simulink model "tp_auto_model (1)"  (R2019a)
settings: Solver=FixedStepAuto  StartTime=0.0  StopTime=20  FixedStep=0.002  RelTol=1e-3  EnableMultiTasking=on
PostLoadFcn:
  | qc_set_target_type(getConfigSet(bdroot, 'QUARC Default Target Configuration'));
values from neighbouring files (symbols this model uses):
  A_c = Axo - L*C    [TP_AUTO_II.m]
  Axo = [ 0 0 1 0 ; 0 0 0 1 ; 0 149 -17 4.91 ; 0 -262 16.8 -8.61]    [TP_AUTO_II.m]
  B_c = [L  Bxo]    [TP_AUTO_II.m]
  Bxo = [0 ; 0 ; -49.7 ; 49.1]    [TP_AUTO_II.m]
  K1 = lqr(Axo , Bxo , Q1 , R)    [TP_AUTO_II.m]
undefined symbols (not defined in the file or in its folder): HIL
libraries: quarc_library x5, cstblocks x2, simulink x1
settings Model: ExtModeTrigDuration=10000  Creator=MLevis  LastModifiedBy=3700500
settings SolverCC: PositivePriorityOrder=on
settings DataIOCC: LimitDataPoints=on  SaveFormat=Array  SignalLoggingSaveFormat=ModelDataLogs  ReturnWorkspaceOutputs=off
settings OptimizationCC: ExpressionDepthLimit=2147483647  InitFltsAndDblsToZero=on  LifeSpan=inf
settings DebuggingCC: SaveWithParameterizedLinksMsg=none  UnderspecifiedInitializationDetection=Classic  MergeDetectMultiDrivingBlocksExec=none  SolverPrmCheckMsg=warning  MultiTaskDSMMsg=warning  MultiTaskCondExecSysMsg=none  FcnCallInpInsideContextMsg=warning  StateNameClashWarn=warning  SFUnexpectedBacktrackingDiag=warning  SFNoUnconditionalDefaultTransitionDiag=warning  SFExecutionAtInitializationDiag=none  ArithmeticOperatorsInVariantConditions=warning
settings HardwareCC: ProdBitPerPointer=32  ProdBitPerSizeT=32  ProdBitPerPtrDiffT=32  ProdLargestAtomicFloat=None  ProdIntDivRoundTo=Undefined  ProdEndianess=Unspecified  ProdWordSize=32  ProdHWDeviceType=32-bit Generic
settings ModelReferenceCC: PropagateSignalLabelsOutOfModel=off
settings SFSimCC: SimUseLocalCustomCode=off
settings RTWCC: SystemTargetFile=quarc_win64.tlc  TemplateMakefile=quarc_default_tmf  Description=QUARC Win64 Target  RTWUseLocalCustomCode=off
settings CodeAppCC: StateflowObjectComments=on
settings STFCustomTargetCC: TargetPreCompLibLocation=C:\PROGRA~3\QUARC\lib\2019a\win64\release  ConcurrentExecutionCompliant=on  GeneratePreprocessorConditionals=Disable all  CPPClassGenCompliant=on  SystemTargetFile=quarc_win64.tlc
settings GRTTargetCC: TargetPreCompLibLocation=C:\PROGRA~3\QUARC\lib\2019a\win64\release  TargetLangStandard=C89/C90 (ANSI)  ParMdlRefBuildCompliant=off  CompOptLevelCompliant=off  GeneratePreprocessorConditionals=Disable all  CombineOutputUpdateFcns=off  MatFileLogging=off  GRTInterface=on  UseToolchainInfoCompliant=off  ExtMode=on  ExtModeMexFile=quarc_comm
settings ConfigComp: CovMetricSettings=dw  CovHtmlReporting=on  CovSaveCumulativeToWorkspaceVar=on  CovSaveSingleToWorkspaceVar=on  CovExternalEMLEnable=off

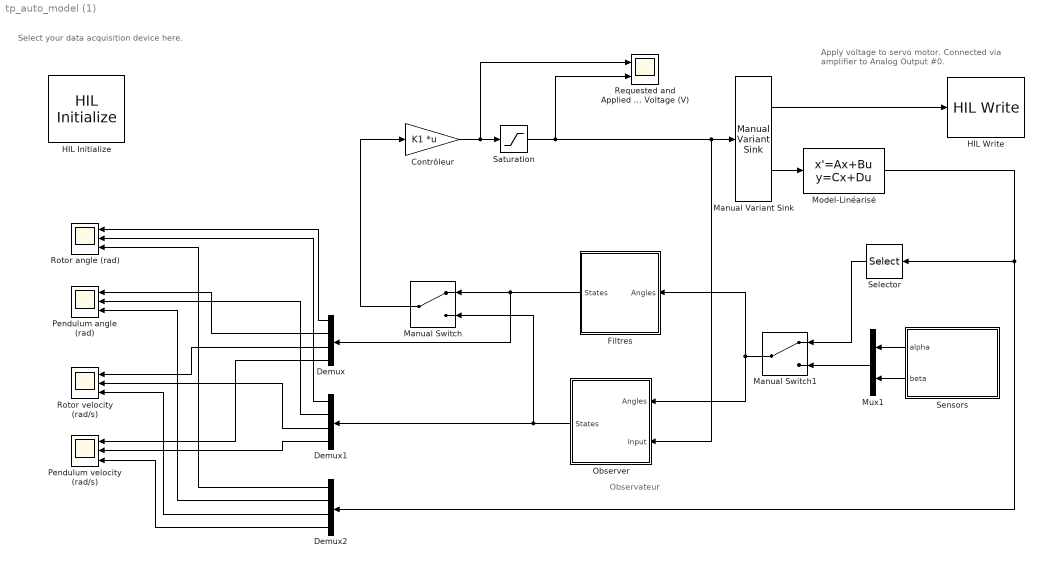
== system tp_auto_model (1) ==
  note: Observateur
  note: Apply voltage to servo motor.
      | Connected via amplifier to Analog Output #0.
  note: Select your data acquisition device here.
  Contrôleur : Gain  Gain=K1  Multiplication=Matrix(K*u) (u vector)
  Demux : Demux
  Demux1 : Demux
  Demux2 : Demux
  "Filtres " : Subsystem
  HIL Initialize : quarc_library/Data Acquisition/Generic/Configuration/HIL Initialize  object_name=HIL-1  board_type=qube_servo2_usb  board_number=0  board_options=""  exclusive=off  active=off  hardware_clocks=[0]  clock_modes=[]  initial_clock_frequencies=[]  set_clock_params_at_start=off  set_clock_params_at_switch_in=off  set_clock_frequencies_at_start=off  set_clock_frequencies_at_switch_in=off  analog_input_channels=[0]  analog_input_configurations=[]  analog_input_maximums=3  analog_input_minimums=-3  set_analog_input_params_at_start=off  set_analog_input_params_at_switch_in=off  analog_output_channels=[0]  analog_output_maximums=15  analog_output_minimums=-15  initial_analog_outputs=[0]  final_analog_outputs=[0]  watchdog_analog_outputs=0  set_analog_output_params_at_start=off  set_analog_output_params_at_switch_in=off  set_analog_outputs_at_start=on  set_analog_outputs_at_switch_in=off  set_analog_outputs_at_terminate=on  set_analog_outputs_at_switch_out=off  set_analog_outputs_on_watchdog=on  digital_input_channels=[]  digital_output_channels=[0]  digital_output_configuration=[]  initial_digital_outputs=[1]  final_digital_outputs=[0]  watchdog_digital_outputs=[0]  set_digital_output_params_at_start=off  set_digital_output_params_at_switch_in=off  set_digital_outputs_at_start=on  set_digital_outputs_at_switch_in=off  set_digital_outputs_at_terminate=on  set_digital_outputs_at_switch_out=off  set_digital_outputs_on_watchdog=on  encoder_channels=[0:1]  quadrature=[4]  encoder_filter_frequency=[]  initial_encoder_counts=[0]  set_encoder_params_at_start=off  set_encoder_params_at_switch_in=off  set_encoder_counts_at_start=on  set_encoder_counts_at_switch_in=off  pwm_channels=[]  pwm_modes=[]  pwm_frequency=[]  pwm_configuration=[]  pwm_alignment=[]  pwm_polarity=[]  pwm_leading_deadband=[]  pwm_trailing_deadband=[]  initial_pwm_outputs=[]  final_pwm_outputs=[]  watchdog_pwm_outputs=[]  set_pwm_params_at_start=off  set_pwm_params_at_switch_in=off  set_pwm_outputs_at_start=off  set_pwm_outputs_at_switch_in=off  set_pwm_outputs_at_terminate=off  set_pwm_outputs_at_switch_out=off  set_pwm_outputs_on_watchdog=off  other_output_channels=[11000:11002]  initial_other_outputs=[0 1 0]  final_other_outputs=[1 0 0]  watchdog_other_outputs=[0 0 1]  set_other_outputs_at_start=on  set_other_outputs_at_switch_in=off  set_other_outputs_at_terminate=on  set_other_outputs_at_switch_out=off  set_other_outputs_on_watchdog=on
  HIL Write : quarc_library/Data Acquisition/Generic/Immediate I//O/HIL Write  Tag=unassigned  object_name=HIL-1  analog_channels=0  pwm_channels=[]  digital_channels=[]  other_channels=[]  sample_time=-1  active=off  vector_input=off
  Manual Variant Sink : simulink/Signal Routing/Manual Variant Sink  NumChoices=2  LabelModeActiveChoice=V_2
      settings: SourceProductName=Simulink
  Manual Switch : ManualSwitch
  Manual Switch1 : ManualSwitch
  Model-Linéarisé : StateSpace  A=Axo  B=Bxo  C=eye(4,4)  D=zeros(4,1)  InitialCondition=[0,pi/2,0,0]
  Mux1 : Mux  Inputs=2
  Observer : Subsystem
  Pendulum angle (rad) : Scope  NumInputPorts=3
  Pendulum velocity (rad/s) : Scope  NumInputPorts=3
  Requested and Applied Motor Voltage (V) : Scope  NumInputPorts=2
  Rotor angle (rad) : Scope  NumInputPorts=3
  Rotor velocity (rad/s) : Scope  NumInputPorts=3
  Saturation : Saturate  UpperLimit=5  LowerLimit=-5
  Selector : Selector  InputPortWidth=4  IndexOptions=Index vector (dialog)  Indices=[1 2]  OutputSizes=1
  "Sensors " : Subsystem
  wires:
  Saturation/1 -> Requested and Applied Motor Voltage (V)/2, Observer/2(Input), Manual Variant Sink/1
  Contrôleur/1 -> Requested and Applied Motor Voltage (V)/1, Saturation/1
  "Sensors "/1(alpha) -> Mux1/1
  "Sensors "/2(beta) -> Mux1/2
  Manual Switch/1 -> Contrôleur/1
  "Filtres "/1(States) -> Demux/1, Manual Switch/1
  Demux/1 -> Rotor angle (rad)/1
  Demux/2 -> Pendulum angle (rad)/1
  Demux/3 -> Rotor velocity (rad/s)/1
  Demux/4 -> Pendulum velocity (rad/s)/1
  Observer/1(States) -> Manual Switch/2, Demux1/1
  Demux1/1 -> Rotor angle (rad)/2
  Demux1/2 -> Pendulum angle (rad)/2
  Demux1/3 -> Rotor velocity (rad/s)/2
  Demux1/4 -> Pendulum velocity (rad/s)/2
  Manual Variant Sink/1 -> HIL Write/1
  Manual Variant Sink/2 -> Model-Linéarisé/1
  Mux1/1 -> Manual Switch1/2
  Manual Switch1/1 -> Observer/1(Angles), "Filtres "/1(Angles)
  Model-Linéarisé/1 -> Demux2/1, Selector/1
  Selector/1 -> Manual Switch1/1
  Demux2/1 -> Rotor angle (rad)/3
  Demux2/2 -> Pendulum angle (rad)/3
  Demux2/3 -> Rotor velocity (rad/s)/3
  Demux2/4 -> Pendulum velocity (rad/s)/3

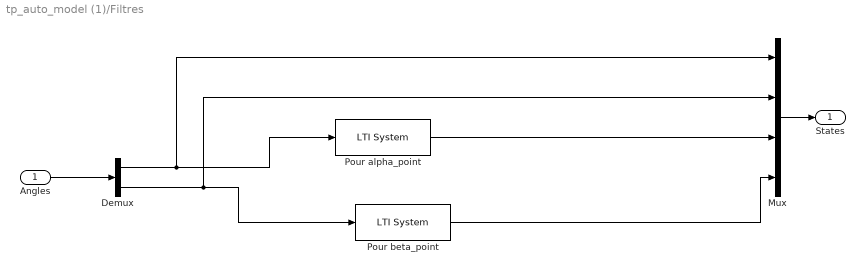
== system tp_auto_model (1)/Filtres  ==
  Angles : Inport
  Demux : Demux  Outputs=2
  Mux : Mux
  Pour alpha_point : cstblocks/LTI System  sys=Filtre_a  IC=[]
  "Pour beta_point " : cstblocks/LTI System  sys=Filtre_b  IC=[]
  States : Outport  VectorParamsAs1DForOutWhenUnconnected=on
  wires:
  Angles/1 -> Demux/1
  Demux/1 -> Pour alpha_point/1, Mux/1
  Demux/2 -> "Pour beta_point "/1, Mux/2
  Mux/1 -> States/1
  Pour alpha_point/1 -> Mux/3
  "Pour beta_point "/1 -> Mux/4

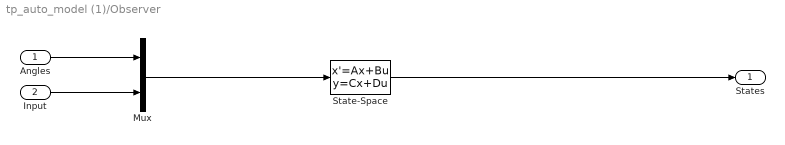
== system tp_auto_model (1)/Observer ==
  Angles : Inport
  Input : Inport  Port=2
  Mux : Mux  Inputs=2
  State-Space : StateSpace  A=A_c  B=B_c  C=eye(4)  D=zeros(4,3)  InitialCondition=[0,0,0,0]
  States : Outport  VectorParamsAs1DForOutWhenUnconnected=on
  wires:
  Angles/1 -> Mux/1
  State-Space/1 -> States/1
  Input/1 -> Mux/2
  Mux/1 -> State-Space/1

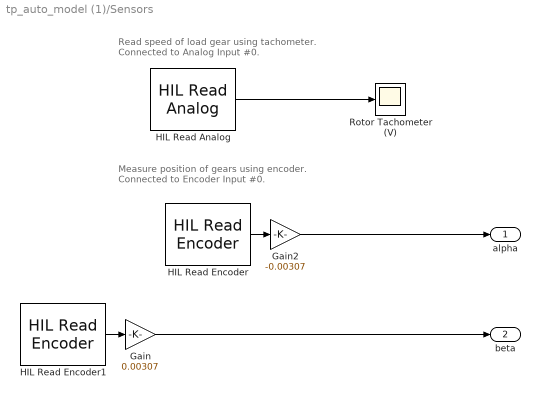
== system tp_auto_model (1)/Sensors  ==
  note: Measure position of gears using encoder.
      | Connected to Encoder Input #0.
  note: Read speed of load gear using tachometer.
      | Connected to Analog Input #0.
  Gain : Gain  Gain=0.00307
  Gain2 : Gain  Gain=-0.00307
  HIL Read Analog : quarc_library/Data Acquisition/Generic/Immediate I//O/HIL Read Analog  object_name=HIL-1  channels=[0]  sample_time=qc_get_step_size  active=on  vector_output=off
  HIL Read Encoder : quarc_library/Data Acquisition/Generic/Immediate I//O/HIL Read Encoder  object_name=HIL-1  channels=0  sample_time=qc_get_step_size  active=on  vector_output=off  data_type_mode=Inherit via back propagation  data_type=double
  HIL Read Encoder1 : quarc_library/Data Acquisition/Generic/Immediate I//O/HIL Read Encoder  object_name=HIL-1  channels=[1]  sample_time=qc_get_step_size  active=on  vector_output=off  data_type_mode=Inherit via back propagation  data_type=double
  Rotor Tachometer (V) : Scope
  alpha : Outport  VectorParamsAs1DForOutWhenUnconnected=on
  beta : Outport  Port=2  VectorParamsAs1DForOutWhenUnconnected=on
  wires:
  Gain2/1 -> alpha/1
  HIL Read Encoder/1 -> Gain2/1
  HIL Read Analog/1 -> Rotor Tachometer (V)/1
  HIL Read Encoder1/1 -> Gain/1
  Gain/1 -> beta/1
